simulink model "engine_throttle"  (R2013b)
settings: Solver=FixedStepDiscrete  StartTime=0  StopTime=1  FixedStep=Ts  RelTol=1e-3
values from neighbouring files (symbols this model uses):
  B = 8.27652280568    [ith_parameter_config.mat]
  J = 0.289072836132    [ith_parameter_config.mat]
  K_ITH_POS_OFFSET = 0    [ith_parameter_config.mat]
  K_ITH_POS_PHYS_K = 32.75    [ith_parameter_config.mat]
  K_ITH_POS_PHYS_OFFSET = 574    [ith_parameter_config.mat]
  Kemf = 0.409607180521    [ith_parameter_config.mat]
  Ksp = 35.4452014593    [ith_parameter_config.mat]
  Kt = 291.958711155    [ith_parameter_config.mat]
  L = 0.30501560014    [ith_parameter_config.mat]
  R = 30.1778654055    [ith_parameter_config.mat]
  springTorqueCompensation = 0    [ith_parameter_config.mat]
  Ts = 0.001    [ith_parameter_config.mat]
undefined symbols (not defined in the file or in its folder): DiscIntNeverNeededParam, rad_init, rad_open, rad_relaxed
settings Model: MinMaxOverflowLogging=MinMaxAndOverflow  FPTRunName=FPA 参照  TunableVars=K_ITH_POS_OFFSET,K_ITH_POS_PHYS_K,K_ITH_POS_PHYS_OFFSET,Ksp,rad_init,rad_open,rad_relaxed,springTorqueCompensation  TunableVarsStorageClass=Auto,Auto,Auto,Auto,Auto,Auto,Auto,Auto  TunableVarsTypeQualifier=,,,,,,,  Creator=The MathWorks Inc.  LastModifiedBy=TTI1783
settings DataIOCC: ExternalInput=[time3,input3]  LimitDataPoints=off  SignalLoggingSaveFormat=ModelDataLogs  SaveOutput=off  SaveTime=off
settings OptimizationCC: InlineParams=on  UseFloatMulNetSlope=on  UseSpecifiedMinMax=on  InlineInvariantSignals=on  EnhancedBackFolding=on  ExpressionDepthLimit=2147483647  ZeroExternalMemoryAtStartup=off  ZeroInternalMemoryAtStartup=off  EfficientFloat2IntCast=on  OptimizeModelRefInitCode=on  LifeSpan=1  BufferReusableBoundary=off
settings DebuggingCC: SignalRangeChecking=warning  SaveWithParameterizedLinksMsg=none  MergeDetectMultiDrivingBlocksExec=error  SolverPrmCheckMsg=none  MultiTaskDSMMsg=warning  MultiTaskCondExecSysMsg=none  ParameterDowncastMsg=warning  ParameterOverflowMsg=warning  ParameterPrecisionLossMsg=none  FcnCallInpInsideContextMsg=UseLocalSettings  BusObjectLabelMismatch=none  StateNameClashWarn=warning  StrictBusMsg=ErrorOnBusTreatedAsVector  LoggingUnavailableSignals=none
settings HardwareCC: ProdLargestAtomicInteger=Long  ProdLargestAtomicFloat=Double  ProdIntDivRoundTo=Floor  ProdEndianess=LittleEndian  ProdHWDeviceType=ARM Compatible->ARM Cortex
settings RTWCC: SystemTargetFile=ert.tlc  GenCodeOnly=on  GenerateMakefile=off  TemplateMakefile=ert_default_tmf  Description=Embedded Coder  GenerateReport=on  ProcessScript=ert_make_rtw_hook  BuildConfiguration=Faster Runs  IncludeHyperlinkInReport=on  LaunchReport=on  IncludeERTFirstTime=on  GenerateTraceInfo=on  GenerateTraceReport=on  GenerateTraceReportSl=on  GenerateTraceReportSf=on  GenerateTraceReportEml=on  RTWCompilerOptimization=On
settings CodeAppCC: ForceParamTrailComments=on  IgnoreCustomStorageClasses=off  IgnoreTestpoints=on  OperatorAnnotations=on  SimulinkDataObjDesc=on  SFDataObjDesc=on  MATLABFcnDesc=on  InsertBlockDesc=on  MATLABSourceComments=on  EnableCustomComments=on  ReqsInCode=on
settings ERTTargetCC: CodeReplacementLibrary=ANSI_C  GenerateSampleERTMain=on  IncludeMdlTerminateFcn=off  CombineSignalStateStructs=on  SuppressErrorStatus=on  SupportNonFinite=off  ERTCustomFileTemplate=example_file_process.tlc  ConvertIfToSwitch=on  SuppressUnreachableDefaultCases=on

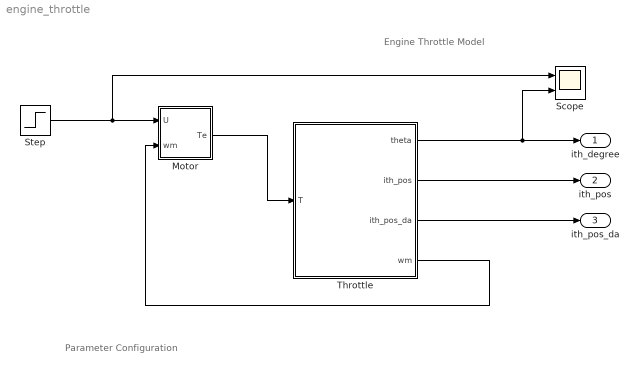
== system engine_throttle ==
  note: Parameter
      | Configuration
  note: Engine Throttle Model
  Motor : Subsystem
  Scope : Scope  NumInputPorts=2
      settings: YMin=-5~-5  YMax=5~5
  Step : Step  Time=.5  Before=12  After=-12  SampleTime=0
  Throttle : Subsystem
  ith_degree : Outport
  ith_pos : Outport  Port=2
  ith_pos_da : Outport  Port=3
  wires:
  Throttle/1(theta) -> Scope/2, ith_degree/1
  Motor/1(Te) -> Throttle/1(T)
  Throttle/2(ith_pos) -> ith_pos/1
  Throttle/4(wm) -> Motor/2(wm)
  Throttle/3(ith_pos_da) -> ith_pos_da/1
  Step/1 -> Scope/1, Motor/1(U)

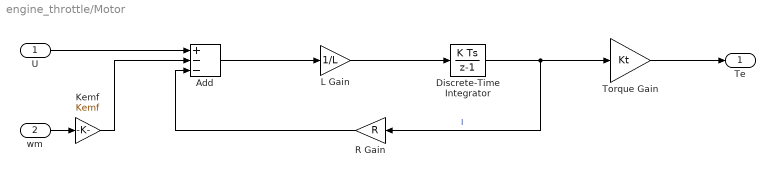
== system engine_throttle/Motor ==
  U : Inport
  wm : Inport  Port=2
  Add : Sum  Inputs=+--  OutDataTypeStr=fixdt(1,32,26)
  Discrete-Time Integrator : DiscreteIntegrator  SampleTime=Ts  OutDataTypeStr=fixdt(1,32,22)  ICPrevOutput=DiscIntNeverNeededParam  ICPrevScaledInput=DiscIntNeverNeededParam
  Kemf : Gain  Gain=Kemf  OutDataTypeStr=fixdt(1,32,28)
  L Gain : Gain  Gain=1/L  OutDataTypeStr=fixdt(1,32,24)
  R Gain : Gain  Gain=R  OutDataTypeStr=fixdt(1,32,26)
  Torque Gain : Gain  Gain=Kt  OutDataTypeStr=fixdt(1,32,23)  ParamDataTypeStr=Inherit: Same as input
  Te : Outport
  wires:
  Add/1 -> L Gain/1
  L Gain/1 -> Discrete-Time Integrator/1
  wm/1 -> Kemf/1
  Kemf/1 -> Add/2
  R Gain/1 -> Add/3
  Discrete-Time Integrator/1 -> Torque Gain/1, R Gain/1  "I"
  Torque Gain/1 -> Te/1
  U/1 -> Add/1

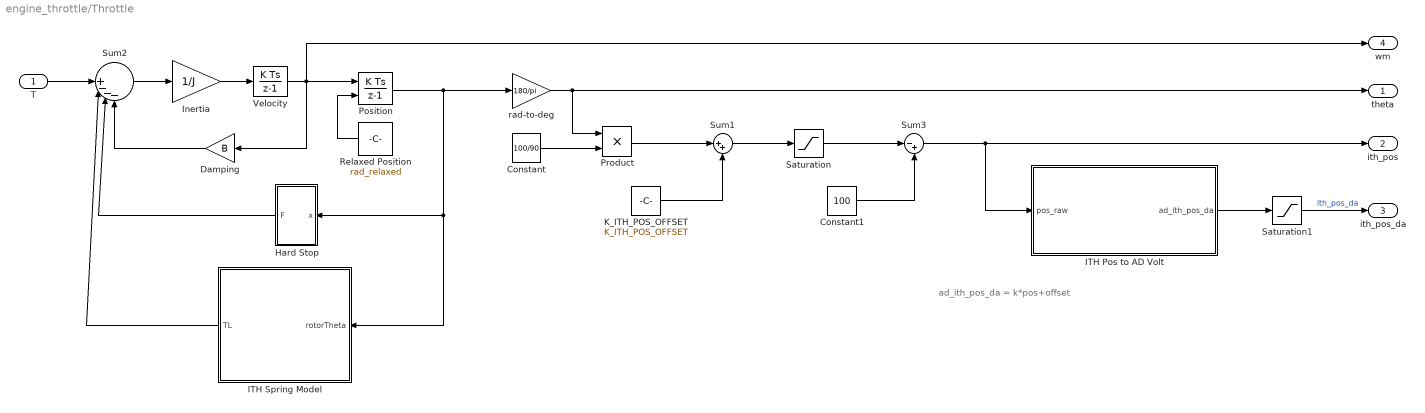
== system engine_throttle/Throttle ==
  note: ad_ith_pos_da = k*pos+offset
  T : Inport
  Constant : Constant  Value=100/90  OutDataTypeStr=fixdt(1,32,30)
  Constant1 : Constant  Value=100  OutDataTypeStr=fixdt(1,32,24)
  Damping : Gain  Gain=B  OutDataTypeStr=fixdt(1,32,23)
  Hard Stop : Subsystem
  ITH Pos to AD Volt : Subsystem
  ITH Spring Model : Subsystem  MinMaxOverflowLogging=MinMaxAndOverflow
  Inertia : Gain  Gain=1/J  OutDataTypeStr=fixdt(1,32,17)  ParamDataTypeStr=Inherit: Same as input
  K_ITH_POS_OFFSET : Constant  Value=K_ITH_POS_OFFSET  OutDataTypeStr=fixdt(1,32,13)
  Position : DiscreteIntegrator  InitialConditionSource=external  SampleTime=Ts  OutDataTypeStr=fixdt(1,32,30)  ICPrevOutput=DiscIntNeverNeededParam  ICPrevScaledInput=DiscIntNeverNeededParam
  Product : Product  OutDataTypeStr=fixdt(1,32,24)
  Relaxed Position : Constant  Value=rad_relaxed  OutDataTypeStr=fixdt(1,32,30)
  Saturation : Saturate  UpperLimit=125  LowerLimit=-25  OutDataTypeStr=fixdt(1,32,24)
  Saturation1 : Saturate  UpperLimit=4095  LowerLimit=0  OutDataTypeStr=fixdt(0,16,4)
  Sum1 : Sum  Inputs=|++  OutDataTypeStr=fixdt(1,32,24)
  Sum2 : Sum  Inputs=|||+---  OutDataTypeStr=fixdt(1,32,18)  SaturateOnIntegerOverflow=on
  Sum3 : Sum  Inputs=|-+  OutDataTypeStr=fixdt(1,32,24)
  Velocity : DiscreteIntegrator  SampleTime=Ts  OutDataTypeStr=fixdt(1,32,26)  ICPrevOutput=DiscIntNeverNeededParam  ICPrevScaledInput=DiscIntNeverNeededParam
  rad-to-deg : Gain  Gain=180/pi  OutDataTypeStr=fixdt(1,32,24)
  theta : Outport
  ith_pos : Outport  Port=2
  ith_pos_da : Outport  Port=3
  wm : Outport  Port=4
  wires:
  Sum3/1 -> ith_pos/1, ITH Pos to AD Volt/1(pos_raw)
  Saturation/1 -> Sum3/1
  Constant1/1 -> Sum3/2
  ITH Spring Model/1(TL) -> Sum2/2
  Hard Stop/1(F) -> Sum2/3
  Saturation1/1 -> ith_pos_da/1  "ith_pos_da"
  K_ITH_POS_OFFSET/1 -> Sum1/2
  Sum1/1 -> Saturation/1
  Product/1 -> Sum1/1
  ITH Pos to AD Volt/1(ad_ith_pos_da) -> Saturation1/1
  Constant/1 -> Product/2
  Relaxed Position/1 -> Position/2
  rad-to-deg/1 -> theta/1, Product/1
  T/1 -> Sum2/1
  Velocity/1 -> Position/1, wm/1, Damping/1
  Inertia/1 -> Velocity/1
  Sum2/1 -> Inertia/1
  Position/1 -> rad-to-deg/1, Hard Stop/1(x), ITH Spring Model/1(rotorTheta)
  Damping/1 -> Sum2/4

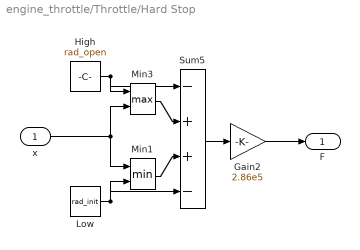
== system engine_throttle/Throttle/Hard Stop ==
  x : Inport
  Gain2 : Gain  Gain=2.86e5  OutDataTypeStr=fixdt(1,32,18)  ParamDataTypeStr=Inherit: Same as input
  High : Constant  Value=rad_open  OutDataTypeStr=fixdt(1,32,30)
  Low : Constant  Value=rad_init  OutDataTypeStr=fixdt(1,32,13)
  Min1 : MinMax  Inputs=2  OutDataTypeStr=fixdt(1,32,30)  SaturateOnIntegerOverflow=on
  Min3 : MinMax  Function=max  Inputs=2  OutDataTypeStr=fixdt(1,32,30)  SaturateOnIntegerOverflow=on
  Sum5 : Sum  Inputs=-+||+-  OutDataTypeStr=fixdt(1,32,12)  SaturateOnIntegerOverflow=on
  F : Outport
  wires:
  Sum5/1 -> Gain2/1
  x/1 -> Min3/2, Min1/1
  Gain2/1 -> F/1
  Min3/1 -> Sum5/2
  Low/1 -> Sum5/4, Min1/2
  High/1 -> Min3/1, Sum5/1
  Min1/1 -> Sum5/3

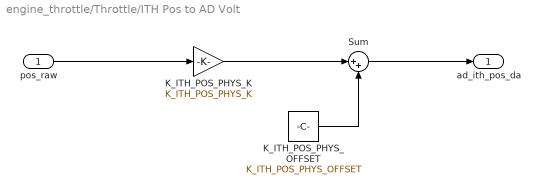
== system engine_throttle/Throttle/ITH Pos to AD Volt ==
  pos_raw : Inport
  K_ITH_POS_PHYS_K : Gain  Gain=K_ITH_POS_PHYS_K  OutDataTypeStr=fixdt(1,32,19)
  K_ITH_POS_PHYS_OFFSET : Constant  Value=K_ITH_POS_PHYS_OFFSET  OutDataTypeStr=fixdt(1,32,21)
  Sum : Sum  Inputs=|++  OutDataTypeStr=fixdt(1,32,19)
  ad_ith_pos_da : Outport
  wires:
  K_ITH_POS_PHYS_K/1 -> Sum/1
  K_ITH_POS_PHYS_OFFSET/1 -> Sum/2
  Sum/1 -> ad_ith_pos_da/1
  pos_raw/1 -> K_ITH_POS_PHYS_K/1

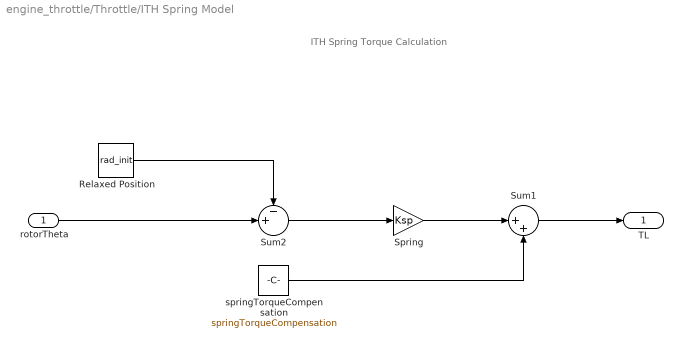
== system engine_throttle/Throttle/ITH Spring Model ==
  note: ITH Spring Torque Calculation
  rotorTheta : Inport
  Relaxed Position : Constant  Value=rad_init  OutDataTypeStr=fixdt(1,32,13)
  Spring : Gain  Gain=Ksp  OutDataTypeStr=fixdt(1,32,25)
  Sum1 : Sum  Inputs=|++  OutDataTypeStr=fixdt(1,32,25)
  Sum2 : Sum  Inputs=-+|  OutDataTypeStr=fixdt(1,32,30)
  springTorqueCompensation : Constant  Value=springTorqueCompensation  OutDataTypeStr=fixdt(1,32,13)
  TL : Outport
  wires:
  Spring/1 -> Sum1/1
  Sum1/1 -> TL/1
  springTorqueCompensation/1 -> Sum1/2
  rotorTheta/1 -> Sum2/2
  Sum2/1 -> Spring/1
  Relaxed Position/1 -> Sum2/1
